simulink model "constraints_comparison_Corsair"  (R2016a)
settings: Solver=ode4  StartTime=0.0  StopTime=30  FixedStep=0.01  RelTol=1e-3
undefined symbols (not defined in the file): acm_aero_model, acm_T_N, breakpoints1, Cm0, Cmde, Cmq, dail, de, dele, drud, Fr_mp_1, Fr_mp_2, Fr_rp_1, Fr_rp_2, ini_acm_de_deg, ini_acm_p_deg_per_s, ini_acm_phi_deg, ini_acm_psi_deg, ini_acm_q_deg_per_s, ini_acm_r_deg_per_s, ini_acm_theta_deg, ini_cmp_de_deg, ini_rig_p_deg_per_s, ini_rig_phi_deg, ini_rig_psi_deg, ini_rig_q_deg_per_s, ini_rig_r_deg_per_s, ini_rig_theta_deg, K1_svo_acm, K1_svo_cmp, K2_svo_acm, K2_svo_cmp, La, Ma, max_defl_sat_acm, max_defl_sat_cmp, max_rate_sat, max_rate_sat_acm, max_rate_sat_cmp, Na, sigbuilder_block, simstop, windspeed, Xa, Ya, Za
libraries: aerolibconvert2 x98, simulink x46, aerolibtransform2 x18
(part 5 of 6)

== matlab function constraints_comparison_Corsair/Equations of motion ==
  data: qa input size=[7,1]; qa_dot_dot output size=[7,1]; qa_dot input size=[7,1]; qa_dot_dot2 input size=[7,1]; theta input; phi input; dail input size=[1,1]; dele input size=[1,1]; drud input size=[1,1]; thrust input; Fa output size=[3,1]; V output; corsair_long output size=[3,1]; corsair_lat output
function [qa_dot_dot, Fa, V, corsair_long,corsair_lat] = fcn(qa, qa_dot, qa_dot_dot2,theta,phi, dail, dele, drud, thrust)

%% Choose constraint type:
% 1 = unconstrained
% 2 = spherical constraint
% 3 = planar constraint

cons = 1;

%% Constants
g = 9.81*0;

% %% Aircraft properties (Hawk)
% 
% m_a = 1.970; % 1.645; % kg
% Ixx_a = 0.008083; % 0.00959; % kg.m^2
% Iyy_a = 0.038; %0.047642; % 0.044; % kg.m^2
% Izz_a = 0.061206; % 0.0507; % kg.m^2
% Ixy_a = 0; % kg.m^2
% Ixz_a = 0; % kg.m^2
% Iyz_a = 0; % kg.m^2
% 
% % Position of body axes origin (c.g. position) relative to inertial axes origin in body frame of reference
% ua0 = [ 0.8*0
%         0.0
%         0.0  ];

%% Aircraft properties (Corsair, taken from Aircraft Stability and Control Data, Gary L. Teper, 1969)

% m_a = 9928.6834; % kg
% Ixx_a = 18486.5777; % kg.m^2
% Iyy_a = 79947.1611; % kg.m^2
% Izz_a = 91599.0606; % kg.m^2
% Ixy_a = 0; % kg.m^2
% Ixz_a = 0; % kg.m^2
% Iyz_a = 0; % kg.m^2

% DC-8
m_a = 86104.03; % kg
Ixx_a = 4216593.82; % kg.m^2
Iyy_a = 3986104.77; % kg.m^2
Izz_a = 7972209.54; % kg.m^2
Ixy_a = -87450.2577; % kg.m^2
Ixz_a = 0; % kg.m^2
Iyz_a = 0; % kg.m^2

% Position of body axes origin (c.g. position) relative to inertial axes origin in body frame of reference
ua0 = [ 0.8*0
        0.0
        0.0  ];
    
%% Input position and attitude vectors

Ra1 = qa(1);
Ra2 = qa(2);
Ra3 = qa(3);
qa0 = qa(4);
qa1 = qa(5);
qa2 = qa(6);
qa3 = qa(7);

%% Input linear and angular velocity vectors

Ra1_dot = qa_dot(1);
Ra2_dot = qa_dot(2);
Ra3_dot = qa_dot(3);
qa0_dot = qa_dot(4);
qa1_dot = qa_dot(5);
qa2_dot = qa_dot(6);
qa3_dot = qa_dot(7);

%% Transformation matrices
            
Ea = [  -qa1     qa0      -qa3     qa2
        -qa2     qa3      qa0      -qa1
        -qa3     -qa2     qa1      qa0  ];
    
E_dasha = [     -qa1     qa0      qa3      -qa2
                -qa2     -qa3     qa0      qa1
                -qa3     qa2      -qa1     qa0  ];
            
Aa = Ea*transpose(E_dasha);

%% Mass and inertial matrix (M) of system
        
% Mass matrix of aircraft model
Ma_RR = [   m_a	0   0
            0   m_a	0
            0   0   m_a	];
        
% Inertial tensor of aircraft model in body frame of reference about c.g./body axes
Ia = [   Ixx_a	-Ixy_a	-Ixz_a
        -Ixy_a	 Iyy_a	-Iyz_a
        -Ixz_a	-Iyz_a	 Izz_a	];
    
MMa = [  Ma_RR    	zeros(3,4)
        zeros(4,3)	transpose(2*E_dasha)*Ia*2*E_dasha	];
    
M = [   MMa  	];

%% Aerodynamics model

rho = 1.225;%1.218; % Density (kg/m^3)
% rho = 1.218; % Density (kg/m^3) Bristol

V_t = 96.6216; %30; % Tunnel windspeed (m/s)

% Calculating angle of attack (alpha), sideslip (sideslip) and local angular velocities (p, q, r)

% Velocity of aircraft in inertial axes
V_a_dot_inertial = [    qa_dot(1)+V_t
                        qa_dot(2)
                        qa_dot(3)      ];
                    
V_a_dot_inertial_pert = [  	qa_dot(1)
                            qa_dot(2)
                            qa_dot(3)      ];
                    
% Acceleration of aircraft in inertial axes (total accelerations is the same are perturbation accelerations)
V_a_dot_dot_inertial_pert = [ 	qa_dot_dot2(1)
                                qa_dot_dot2(2)
                                qa_dot_dot2(3)   ];

% Velocity of aircraft in body axes (vector_inertial = A * vector_body, where A is the transformation matrix)
V_a_dot_body = transpose(Aa)*V_a_dot_inertial;
V_a_dot_body_pert = transpose(Aa)*V_a_dot_inertial_pert;

% Acceleration of aircraft in body axes (vector_inertial = A * vector_body, where A is the transformation matrix)
V_a_dot_dot_body_pert = transpose(Aa)*V_a_dot_dot_inertial_pert;

% Magnitude of total local velocity vector
V = sqrt((V_a_dot_inertial(1))^2+(V_a_dot_inertial(2))^2+(V_a_dot_inertial(3))^2);

% Angle of attack (alpha)
alpha = atan2(V_a_dot_body(3),V_a_dot_body(1));

% Sideslip angle (beta)
beta = asin(V_a_dot_body(2)/V);

% Local angular velocities (p, q, r in body axes)
omega_dasha = 2*E_dasha*[	qa0_dot
                            qa1_dot
                            qa2_dot
                            qa3_dot     ];

p = omega_dasha(1);
q = omega_dasha(2);
r = omega_dasha(3);

% % Reference dimensions (Hawk)
% c = 0.143;        % m
% S = 0.084942;     % m^2
% b = 0.594;        % m
% Reference dimensions (Corsair, taken from Aircraft Stability and Control Data, Gary L. Teper, 1969)
c = 3.29184;      	% m
S = 33.1664;     	% m^2
b = 11.79576;     	% m

% Reference dimensions (Corsair, taken from Aircraft Stability and Control Data, Gary L. Teper, 1969)
c2 = 3.29184;      	% m
S2 = 33.1664;     	% m^2
b2 = 11.79576;     	% m

% A-7A Corsair II (taken from Aircraft Stability and Control Data, Gary L. Teper, 1969)
% Flight conditions: 15,000 ft at Mach 0.3 (no. 4 in reference)
% Initial angle of attack = 13.3 deg
% Initial elevator deflection = -8.8 deg

rho2 = 0.77100671563;	% kg/m^3 (0.001496 slugs/ft^3)
qbar = 367.6468;        % kg/m^2 (75.3 lb/ft^2)
VT0 = 96.6216;          % m/s (317 ft/sec)
U0 = 94.1832;           % m/s (309 ft/sec)

m_a2 = 9928.6834;       % kg
Ixx_a2 = 18486.5777;    % kg.m^2
Iyy_a2 = 79947.1611; 	% kg.m^2
Izz_a2 = 91599.0606; 	% kg.m^2

% Longitudinal dimensional derivatives (body axes, taken from Aircraft Stability and Control Data, Gary L. Teper, 1969)
% X_w     =   0.00464;    % 1/s
% X_u     =   0.00501;    % 1/s
% X_dele  =   5.63;       % ft/(s^2 rad)
% Z_w     =   -0.545;     % 1/s
% Z_u     =   -0.0857;    % 1/s
% Z_dele  =   -23.8;      % ft/(s^2 rad)
% M_w     =   -0.00777;   % 1/(s ft)
% M_w_dot =   -0.000178;  % 1/(s ft)
% M_q     =   -0.340;     % 1/s
% M_u     =   0.00183;    % 1/(s ft)
% M_dele  =   -4.52;      % 1/s^2
% Longitudinal dimensional derivatives (body axes, taken from Cook page 148)
% X_q     =   -72.9;      % ft/s
% X_theta =   -31.34;     % ft/(s^2 rad)
% Z_q     =   309.0;      % ft/s
% Z_theta =   -7.4;       % ft/(s^2 rad)
% M_q see above
% M_theta =   0.00132;    % 1/s^2

% Units conversion
X_u     =   0.00501;                    % 1/s
X_w     =   0.00464;                    % 1/s
X_q     =   -72.9*0.3048;               % m/s
X_theta =   -31.34*0.3048;              % m/(s^2 rad)
X_dele  =   5.63*0.3048;                % m/(s^2 rad)
Z_u     =   -0.0857;                    % 1/s
Z_w     =   -0.545;                     % 1/s
Z_q     =   309.0*0.3048;               % m/s
Z_theta =   -7.4*0.3048;                % m/(s^2 rad)
Z_dele  =   -23.8*0.3048;               % m/(s^2 rad)
M_u     =   0.00183*(1/0.3048);         % 1/(s m)
M_w     =   -0.00777*(1/0.3048);        % 1/(s m)
% M_w_dot =   -0.000178*(1/0.3048);       % 1/(s m)
M_q     =   -0.340*0-0.395;            	% 1/s
M_theta =   0.00132;                    % 1/s^2
M_dele  =   -4.52;                      % 1/s^2

% % % % Longitudinal dimensional derivatives (body axes, taken from Aircraft Stability and Control Data, Gary L. Teper, 1969)
% % % % Y_v     =   -0.122;       % 1/s
% % % % Y_dail  =   -0.00150;     % ft/(s^2)
% % % % Y_drud  =   0.0307;       % ft/(s^2)
% % % % L_beta  =   -8.79;        % 1/s^2
% % % % L_p     =   -1.38;        % 1/s
% % % % L_r     =   0.857;        % 1/s
% % % % L_dail  =   3.75;         % 1/s^2
% % % % L_drud  =   1.82;         % 1/s^2
% % % % N_beta  =   0.948;        % 1/s^2 
% % % % N_p     =   -0.0310;      % 1/s
% % % % N_r     =   -0.271;       % 1/s     
% % % % N_dail  =   0.280;        % 1/s^2
% % % % N_rud   =   -1.56;        % 1/s^2
% % % 
% % % % Units conversion
% % % Y_v     =   -0.122;             % 1/s
% % % Y_dail  =   -0.00150*0.3048;   	% m/(s^2)
% % % Y_drud  =   0.0307*0.3048;     	% m/(s^2)
% % % L_beta  =   -8.79;              % 1/s^2
% % % L_p     =   -1.38;              % 1/s
% % % L_r     =   0.857;              % 1/s
% % % L_dail  =   3.75;               % 1/s^2
% % % L_drud  =   1.82;               % 1/s^2
% % % N_beta  =   0.948;              % 1/s^2
% % % N_p     =   -0.0310;            % 1/s
% % % N_r     =   -0.271;             % 1/s
% % % N_dail  =   0.280;              % 1/s^2
% % % N_drud   =   -1.56;              % 1/s^2

% Longitudinal dimensional derivatives (body axes, taken from Aircraft Stability and Control Data, Gary L. Teper, 1969)
% Y_v     =   -0.122;       % 1/s
% Y_dail  =   -0.00150;     % ft/(s^2)
% Y_drud  =   0.0307;       % ft/(s^2)
% L_beta  =   -8.79;        % 1/s^2
% L_p     =   -1.38;        % 1/s
% L_r     =   0.857;        % 1/s
% L_dail  =   3.75;         % 1/s^2
% L_drud  =   1.82;         % 1/s^2
% N_beta  =   0.948;        % 1/s^2 
% N_p     =   -0.0310;      % 1/s
% N_r     =   -0.271;       % 1/s     
% N_dail  =   0.280;        % 1/s^2
% N_rud   =   -1.56;        % 1/s^2
% Lateral dimensional derivatives (body axes, taken from Cook page 185)
% Y_phi   =   32.2;         % ft/(s^2 rad)
% Y_r     =   -468.2;       % ft/s

% Units conversion
Y_v     =   -0.1008;                                % 1/s
Y_phi   =   32.2*0.3048;                            % m/(s^2 rad)
Y_r     =   -468.2*0.3048;                          % m/s
Y_dail  =   0*0.3048;                               % m/(s^2)
Y_drud  =   13.48416*0.3048;                        % m/(s^2)
L_v     =   -2.6826/(468.2*0.3048); %-2.71/468.2;  	% 1/s^2
L_p     =   -1.2332; %-1.232;                       % 1/s
L_r     =   0.3913; %0.397;                         % 1/s
L_dail  =   -1.62;                                  % 1/s^2
L_drud  =   0.392;                                  % 1/s^2
N_v     =   1.2710/(468.2*0.3048); %1.301/468.2; 	% 1/s^2
N_p     =   -0.0481; %-0.0346;                    	% 1/s
N_r     =   -0.2524; %-0.257;                       % 1/s
N_dail  =   -0.0365; %-0.01875;                     % 1/s^2
N_drud  =   -0.8602; %-0.864;                       % 1/s^2

% Body axis velocities (p, q, r are already defined above)
u = V_a_dot_body_pert(1);
v = V_a_dot_body_pert(2);
w = V_a_dot_body_pert(3);
% w_dot = V_a_dot_dot_body_pert(3);

% % % % Converting to nondimensional derivatives (see Aircraft Stability and Control Data, Gary L. Teper, 1969)
% % % CX_w     =   X_w*(2*m_a2)/(rho2*S2*U0);
% % % CX_u     =   X_u*(m_a2)/(rho2*S2*U0);
% % % CX_dele  =   -X_dele*(2*m_a2)/(rho2*S2*VT0^2);
% % % CZ_w     =   Z_w*(2*m_a2)/(rho2*S2*U0);
% % % CZ_u     =   Z_u*(m_a2)/(rho2*S2*U0);
% % % CZ_dele  =   -Z_dele*(2*m_a2)/(rho2*S2*VT0^2);
% % % CM_w     =   M_w*(2*Iyy_a2)/(rho2*S2*c2*U0);
% % % CM_w_dot =   M_w_dot*(4*Iyy_a2*VT0)/(rho2*S2*c2^2*U0);
% % % CM_q     =   M_q*(4*Iyy_a2)/(rho2*S2*c2^2*VT0);
% % % CM_u     =   M_u*(2*Iyy_a2)/(rho2*S2*c2*U0);
% % % CM_dele  =   M_dele*(2*Iyy_a2)/(rho2*S2*c2*VT0);
% % % 
% % % CX = -(CX_w*w + CX_u*u + CX_dele*dele); % Negative because Teper sign convention is positive aft
% % % CZ = CZ_w*w + CZ_u*u + CZ_dele*dele;
% % % % CM = CM_w*w + CM_w_dot*w_dot + CM_q*q + CM_u*u + CM_dele*dele;
% % % CM = CM_w*w + CM_q*q + CM_u*u + CM_dele*dele;
% % % 
% % % CY = 0;
% % % CL = 0;
% % % CN = 0;

X_body = m_a*X_w*w + m_a*X_u*u + m_a*X_dele*dele + m_a*X_q*q + m_a*X_theta*theta;
Y_body = m_a*Y_v*v + m_a*Y_dail*dail + m_a*Y_drud*drud + m_a*Y_phi*phi + m_a*Y_r*r;
Z_body = m_a*Z_w*w + m_a*Z_u*u + m_a*Z_dele*dele + m_a*Z_q*q + m_a*Z_theta*theta;

L_body = Ixx_a*L_v*v + Ixx_a*L_p*p + Ixx_a*L_r*r + Ixx_a*L_dail*dail + Ixx_a*L_drud*drud;
M_body = Iyy_a*M_w*w + Iyy_a*M_u*u + Iyy_a*M_dele*dele + Iyy_a*M_q*q + Iyy_a*M_theta*theta;
N_body = Izz_a*N_v*v + Izz_a*N_p*p + Izz_a*N_r*r + Izz_a*N_dail*dail + Izz_a*N_drud*drud;
    
% Wind axes forces and moments
% % % X_wind=0.5*rho*V^2*S*CX;
% % % Y_wind=0.5*rho*V^2*S*CY;
% % % Z_wind=0.5*rho*V^2*S*CZ;
% % % 
% % % L_wind=0.5*rho*V^2*S*b*CL;
% % % M_wind=0.5*rho*V^2*S*c*CM;
% % % N_wind=0.5*rho*V^2*S*b*CN;

% X_wind=0.5*rho2*V^2*S*CX;
% Y_wind=0.5*rho2*V^2*S*CY;
% Z_wind=0.5*rho2*V^2*S*CZ;
% 
% L_wind=0.5*rho2*V^2*S*b*CL;
% M_wind=0.5*rho2*V^2*S*c*CM;
% N_wind=0.5*rho2*V^2*S*b*CN;

% F_wind = [  X_wind
%             Y_wind
%             Z_wind   ];
%         
% M_wind = [  L_wind
%             M_wind
%             N_wind   ];
        
% Body to wind axes transformation
% According to Cook (page 21): (phi,theta,psi) = (0,alpha,-beta)
phi_w = 0;
theta_w = alpha;
psi_w = -beta;

% From NASA transformation equations:
theta1 = psi_w;
theta2 = theta_w;
theta3 = phi_w;

q0 = +sin(theta1/2)*sin(theta2/2)*sin(theta3/2)+cos(theta1/2)*cos(theta2/2)*cos(theta3/2);
q1 = -sin(theta1/2)*sin(theta2/2)*cos(theta3/2)+sin(theta3/2)*cos(theta1/2)*cos(theta2/2);
q2 = +sin(theta1/2)*sin(theta3/2)*cos(theta2/2)+sin(theta2/2)*cos(theta1/2)*cos(theta3/2);
q3 = +sin(theta1/2)*cos(theta2/2)*cos(theta3/2)-sin(theta2/2)*sin(theta3/2)*cos(theta1/2);

E = [  -q1     q0      -q3     q2
        -q2     q3      q0      -q1
        -q3     -q2     q1      q0  ];
    
E_dash = [     -q1     q0      q3      -q2
                -q2     -q3     q0      q1
                -q3     q2      -q1     q0  ];
            
A_b2w = E*transpose(E_dash); % Note: this matrx transforms from body to wind axes!

% Body axes forces and moments
% F_dash_a = transpose(A_b2w)*F_wind + [thrust;0;0];
% M_dash_a = transpose(A_b2w)*M_wind;
F_dash_a = [X_body*0;Y_body;Z_body*0] + [thrust;0;0];
M_dash_a = [L_body;M_body*0;N_body];

% Inertial axes moments
F_a = Aa*F_dash_a;

%% Computing external forces matrix QE
                
% Angular velocity of aircraft model in body frame of reference
omega_dasha = 2*E_dasha*[	qa0_dot
                            qa1_dot
                            qa2_dot
                            qa3_dot     ];
                        
% External translational/linear forces on aircraft model in inertial frame of reference
% Fa1 = 0;
% Fa2 = 0;
% Fa3 = m_a*9.81;
Fa1 = F_a(1);
Fa2 = F_a(2);
Fa3 = F_a(3)+m_a*g;
Fa = [  Fa1
        Fa2
        Fa3    ];
% External moments on aircraft model in body frame of reference
% Ma1 = 0;
% Ma2 = 0;
% Ma3 = 0;
Ma1 = M_dash_a(1);
Ma2 = M_dash_a(2);
Ma3 = M_dash_a(3);
Ma = [  Ma1
        Ma2
        Ma3     ];

QE_a = [    Fa
            transpose(2*E_dasha)*(Ma-cross(omega_dasha,Ia*omega_dasha))	];
        
QE = [  QE_a    ];

%% Solving equations of motion

switch cons
    case 1 % Unconstrained
        
        % Quaternion constriant
        Cq_1 = [	zeros(1,3)	qa0   qa1   qa2   qa3  ];
        QC_1 = -((qa0_dot)^2+(qa1_dot)^2+(qa2_dot)^2+(qa3_dot)^2);
        
        Cq = Cq_1;
        QC = QC_1;
        
    case 2 % Spherical constraint
        
        % Quaternion constriant
        Cq_1 = [	zeros(1,3)	qa0   qa1   qa2   qa3  ];
        QC_1 = -((qa0_dot)^2+(qa1_dot)^2+(qa2_dot)^2+(qa3_dot)^2);
        
        % Spherical constraint
        r = 0.8; % Sphere radius (m)
        Cq_2 = [    (Ra1-r)   Ra2     Ra3     0   0   0   0];
        QC_2 = -Ra1_dot^2 - Ra2_dot^2 - Ra3_dot^2;
        
        Cq = [  Cq_1
                Cq_2  ];
        QC = [  QC_1
                QC_2  ];
        
    case 3 % Planar constraint
        
        % Quaternion constriant
        Cq_1 = [	zeros(1,3)	qa0   qa1   qa2   qa3  ];
        QC_1 = -((qa0_dot)^2+(qa1_dot)^2+(qa2_dot)^2+(qa3_dot)^2);
        
        % Planar constraint
        Cq_2 = [    1   0   0   0   0   0   0   ];
        QC_2 = 0;
        
        Cq = [  Cq_1
                Cq_2  ];
        QC = [  QC_1
                QC_2  ];
            
    case 4 % x and z constriant for validating lateral aerodynamics model
        
        % Quaternion constriant
        Cq_1 = [	zeros(1,3)	qa0   qa1   qa2   qa3  ];
        QC_1 = -((qa0_dot)^2+(qa1_dot)^2+(qa2_dot)^2+(qa3_dot)^2);
        
        % x constraint
        Cq_2 = [    1   0   0   0   0   0   0   ];
        QC_2 = 0;
        
     	% x constraint
        Cq_3 = [    0   0   1   0   0   0   0   ];
        QC_3 = 0;
        
        Cq = [  Cq_1
                Cq_2
                Cq_3  ];
        QC = [  QC_1
                QC_2
                QC_3  ];
        
end

        
MM = [  M   transpose(Cq)
        Cq  zeros(size(QC,1))        ];
QQ = [  QE
        QC  ];

qq = MM\QQ;

%% Output acceleration vectors

qa_dot_dot = qq(1:7);

%% Output for comparing with Cook Corsair model (For theta_a, see output from quaternion converison block)
uu_a        = qa_dot(1)*3.28084; % ft/sec
vv_a        = qa_dot(2)*3.28084; % ft/sec
ww_a        = qa_dot(3)*3.28084; % ft/sec
pp_a        = p;                 % rad/s
qq_a        = q;                 % rad/s
rr_a        = r;                 % rad/s

corsair_long = [ uu_a
                 ww_a
                 qq_a ];
             
corsair_lat  = [ vv_a
                 pp_a
                 rr_a ];

== matlab function constraints_comparison_Corsair/Subsystem14/Subsystem13/MATLAB Function ==
  data: q input; x_ini output; y_ini output; z_ini output
function [x_ini,y_ini,z_ini]= fcn(q)

% Initial position

x = 0.8;
z = 0.1433;%0.03975;

p = [   x
        0
        z   ];

q0 = q(1);
q1 = q(2);
q2 = q(3);
q3 = q(4);

E = [  -q1     q0      -q3     q2
       -q2     q3      q0      -q1
       -q3     -q2     q1      q0  ];
    
E_dash = [     -q1     q0      q3      -q2
               -q2     -q3     q0      q1
               -q3     q2      -q1     q0  ];
           
A = E*transpose(E_dash);

p_in = A*p;

x_ini = p_in(1);
y_ini = p_in(2);
z_ini = p_in(3);

== matlab function constraints_comparison_Corsair/Subsystem14/Aircraft acceleration body axis ==
  data: Aa input; qa_dot_dot3 output; qa_dot_dot2 input; nz output
function [qa_dot_dot3,nz]= fcn(Aa, qa_dot_dot2)

% qa_dot_dot2 = linear accelerations in inertial frame
% qa_dot_dot3 = linear accelerations in body axis

qa_dot_dot3 = Aa\qa_dot_dot2;
% qa_dot_dot3 = qa_dot_dot2;

theta_acm = atan(-Aa(3,1)/sqrt(1-(Aa(3,1))^2));
nz = qa_dot_dot2(3)*cos(theta_acm)-qa_dot_dot2(1)*sin(theta_acm);

== matlab function constraints_comparison_Corsair/Subsystem14/Aerodynamics model: compensator ==
  data: qc input; V_t input; alpha input; beta input; q input; eta input; F_c output; M_dash_c output; r input; rudd input; extra output
function [F_c,M_dash_c,extra] = fcn(qc,V_t,alpha,beta,q,eta,r,rudd)

% beta = 0;

Rc1 = qc(1);
Rc2 = qc(2);
Rc3 = qc(3);
qc0 = qc(4);
qc1 = qc(5);
qc2 = qc(6);
qc3 = qc(7);

% Transformation matrices
Ec = [  -qc1     qc0      -qc3     qc2
        -qc2     qc3      qc0      -qc1
        -qc3     -qc2     qc1      qc0  ];
    
E_dashc = [     -qc1     qc0      qc3      -qc2
                -qc2     -qc3     qc0      qc1
                -qc3     qc2      -qc1     qc0  ];

Ac = Ec*transpose(E_dashc);

% Reference dimensions
c = 0.181;      % m
S = 0.1254;     % m^2
b = 0.7;        % m

% % Control surface deflection
% eta = dcs(1); % Virtual ailerons
% eta = dcs(2); % Virtual elevator
% eta = dcs(3); % Virtual rudder

% Aerodynamic coefficients (alpha = theta_rig)
% CL=3.647*alpha+1.306*eta+(2.302*0.181/V_t)*q; % Pattinson
% CL=2.18*alpha+0.5*eta+(b*15/(2*V_t))*q; % Matthew (old)
CL=1.73*alpha+1.42*eta+(b*4.69/(2*V_t))*q; % Matthew (13th Oct 2015)
% CD=CL^2/(3.907*pi); % Pattinson
CD=0; % Matthew
CM=0; % Pattinson/Matthew

% Side force
CY = 1.73*-beta+1.42*rudd+(b*4.69/(2*V_t))*r;

% Dynamic pressure
rho = 1.225;% 1.218; % Density (kg/m^3)
Dyn_p = 0.5*rho*V_t^2;

% Loads in wind axes (relative to total local velocity vector)
L = Dyn_p*S*CL;
D = Dyn_p*S*CD;
M = Dyn_p*S*c*CM;

Y = Dyn_p*S*CY;

% Transforming loads to body frame of reference from wind axes (See Cook p.21)
phi = 0;
theta = alpha;
psi = -beta;

% q0 = cos(phi/2)*cos(theta/2)*cos(psi/2)+sin(phi/2)*sin(theta/2)*sin(psi/2);
% q1 = cos(phi/2)*cos(theta/2)*sin(psi/2)-sin(phi/2)*sin(theta/2)*cos(psi/2);
% q2 = cos(phi/2)*sin(theta/2)*cos(psi/2)+sin(phi/2)*cos(theta/2)*sin(psi/2);
% q3 = sin(phi/2)*cos(theta/2)*cos(psi/2)-cos(phi/2)*sin(theta/2)*sin(psi/2);
% 
% E = [  -q1     q0      -q3     q2
%         -q2     q3      q0      -q1
%         -q3     -q2     q1      q0  ];
%     
% E_dash = [     -q1     q0      q3      -q2
%                 -q2     -q3     q0      q1
%                 -q3     q2      -q1     q0  ];
%             
% A = E*transpose(E_dash);

theta1 = psi;
theta2 = theta;
theta3 = phi;

q0 = +sin(theta1/2)*sin(theta2/2)*sin(theta3/2)+cos(theta1/2)*cos(theta2/2)*cos(theta3/2);
q1 = -sin(theta1/2)*sin(theta2/2)*cos(theta3/2)+sin(theta3/2)*cos(theta1/2)*cos(theta2/2);
q2 = +sin(theta1/2)*sin(theta3/2)*cos(theta2/2)+sin(theta2/2)*cos(theta1/2)*cos(theta3/2);
q3 = +sin(theta1/2)*cos(theta2/2)*cos(theta3/2)-sin(theta2/2)*sin(theta3/2)*cos(theta1/2);

E = [	-q1     q0      -q3     q2
        -q2     q3      q0      -q1
        -q3     -q2     q1      q0  ];
    
E_dash = [	-q1     q0      q3      -q2
           	-q2     -q3     q0      q1
           	-q3     q2      -q1     q0  ];
            
A10 = E*transpose(E_dash);
A10_transpose_inertial_to_body = A10';

F_dash_c = A10_transpose_inertial_to_body*[ -D
                                            Y
                                            -L  ];
                      
% M_dash_c = transpose(A)*[ 0
%                           M
%                           0   ];
M_dash_c = A10_transpose_inertial_to_body*[  0
                                             M
                                             0   ];
                    
% Transforming forces onto inertial frame
F_c = Ac*F_dash_c;

% F_c = [     -D*0
%             0
%             -L  ]; %/cos(alpha)

% F_c = zeros(3,1);
% M_dash_c = zeros(3,1);

%% Extra
extra = [   alpha*180/pi
            beta*180/pi
            -D
            Y
            -L
            F_dash_c
            F_c];

== matlab function constraints_comparison_Corsair/Subsystem14/MATLAB Function7 ==
  data: V_t output size=[1]; qc input size=[7,1]; theta_rig output size=[1]; p output; qc_dot input size=[7,1]; q output size=[1]; r output; qc_dot_dot input; Vt input; Vc output; omega_dashc_dot output
function [V_t,theta_rig,p,q,r,Vc,omega_dashc_dot] = fcn(qc,qc_dot,qc_dot_dot,Vt)
  
Rc1 = qc(1);
Rc2 = qc(2);
Rc3 = qc(3);
qc0 = qc(4);
qc1 = qc(5);
qc2 = qc(6);
qc3 = qc(7);

Rc1_dot = qc_dot(1);
Rc2_dot = qc_dot(2);
Rc3_dot = qc_dot(3);
qc0_dot = qc_dot(4);
qc1_dot = qc_dot(5);
qc2_dot = qc_dot(6);
qc3_dot = qc_dot(7);

Rc1_dot_dot = qc_dot_dot(1);
Rc2_dot_dot = qc_dot_dot(2);
Rc3_dot_dot = qc_dot_dot(3);
qc0_dot_dot = qc_dot_dot(4);
qc1_dot_dot = qc_dot_dot(5);
qc2_dot_dot = qc_dot_dot(6);
qc3_dot_dot = qc_dot_dot(7);

% Transformation matrices
Ec = [  -qc1     qc0      -qc3     qc2
        -qc2     qc3      qc0      -qc1
        -qc3     -qc2     qc1      qc0  ];
    
E_dashc = [     -qc1     qc0      qc3      -qc2
                -qc2     -qc3     qc0      qc1
                -qc3     qc2      -qc1     qc0  ];

Ac = Ec*transpose(E_dashc);

% Wind tunnel velocity vector
Vtt = [  Vt
         0   
         0   ];

% Velocity vector of aircraft model in inertial frame of reference
Vc = [  Rc1_dot
        Rc2_dot
        Rc3_dot	];

% Total velocity vector of aircraft model in body frame of reference
Vc_dash = transpose(Ac)*(Vc + Vtt);

% Magnitude of total local velocity vector
V0 = sqrt((Vc_dash(1))^2+(Vc_dash(2))^2+(Vc_dash(3))^2);

% Angle of attack
alpha = atan2(Vc_dash(3),Vc_dash(1));

% Acceleration in body frame
c_dash = transpose(Ac)*[    Rc1_dot_dot
                            Rc2_dot_dot
                            Rc3_dot_dot     ];

% Acceleration in z-direction body frame
w_dot = c_dash(3);

% Sideslip angle [CHECK SIGN]
beta = asin(Vc_dash(2)/V0);

% Local angular velocities
omega_dashc = 2*E_dashc*[	qc0_dot
                            qc1_dot
                            qc2_dot
                            qc3_dot     ];
                        
% Angular rate
p = omega_dashc(1); % rad/s
q = omega_dashc(2); % rad/s
r = omega_dashc(3); % rad/s

V_t = Vtt(1);

% Rig pitch angle
% theta_rig = atan2(-Ac(3,1),sqrt(1-(Ac(3,1))^2));
theta_rig = 0;

%% Local angular acceleration
omega_dashc_dot = 2*E_dashc*[	qc0_dot_dot
                            qc1_dot_dot
                            qc2_dot_dot
                            qc3_dot_dot     ];

== matlab function constraints_comparison_Corsair/Subsystem14/Aerodynamics model: Hawk ==
  data: Cm0 input; Cmde input; de input; Cmq input; T input; acm_aero_model input; qa input; V0 input; alpha input; w_dot input; q input; eta input; F_a output; M_dash_a output; q_rig input; Aa output
function [F_a,M_dash_a,Aa] = fcn(Cm0,Cmde,de,Cmq,T,acm_aero_model,qa,V0,alpha,w_dot,q,eta,q_rig)

beta = 0;

Ra1 = qa(1);
Ra2 = qa(2);
Ra3 = qa(3);
qa0 = qa(4);
qa1 = qa(5);
qa2 = qa(6);
qa3 = qa(7);

% Transformation matrices
Ea = [  -qa1     qa0      -qa3     qa2
        -qa2     qa3      qa0      -qa1
        -qa3     -qa2     qa1      qa0  ];
    
E_dasha = [     -qa1     qa0      qa3      -qa2
                -qa2     -qa3     qa0      qa1
                -qa3     qa2      -qa1     qa0  ];

Aa = Ea*transpose(E_dasha);

% Reference dimensions (Hawk)
c = 0.143;       % m
S = 0.084942;    % m^2

% theta_acm = atan(-Aa(3,1)/sqrt(1-(Aa(3,1))^2));
% aplha_approx = theta_acm -0.8*q_rig/30;

% Aerodynamic coefficients
% (Note: CL0=0.1155 is multiplied by a factor of 1.80 to match experimental
%  data)
% CL=0.1155*1.80/1.80+3.8004*alpha+0.4429*eta-0.4456*alpha*eta-4.447*alpha^2-0.04322*eta^2-7.314*alpha*eta^2-4.636*alpha^2*eta+0.0008039*alpha^3+0.001499*eta^3+1.828*q*c/V0*0+33*(c/(2*V0))*q+1.342*c/(V0^2)*w_dot*0;
% CD=0.04953+0.04801*alpha-0.008018*eta+0.4703*alpha*eta+1.669*alpha^2+0.3445*eta^2+0.2102*alpha*eta^2-0.9875*alpha^2*eta+0.00001016*alpha^3-0.00002714*eta^3;
% CM=0.04463-0.5919*alpha-0.7774*eta+0.4383*alpha*eta-0.1227*alpha^2-0.4214*eta^2-2.587*alpha*eta^2+3.292*alpha^2*eta-0.0001252*alpha^3-0.002631*eta^3-3.528*q*c/V0-2.604*c/(V0^2)*w_dot*0;

% CL=0.1155*0.75+3.8004*0.75*alpha+0.4429*0.75*eta-0.4456*alpha*eta-4.447*alpha^2-0.04322*eta^2-7.314*alpha*eta^2-4.636*alpha^2*eta+0.0008039*alpha^3+0.001499*eta^3-1.828*q*c/V0-1.342*c/(V0^2)*w_dot;
% CD=0.04953*0.75+0.04801*0.75*alpha-0.008018*0.75*eta+0.4703*alpha*eta+1.669*alpha^2+0.3445*eta^2+0.2102*alpha*eta^2-0.9875*alpha^2*eta+0.00001016*alpha^3-0.00002714*eta^3;
% CM=0.04463*0.75-0.5919*0.75*alpha-0.7774*0.75*eta+0.4383*alpha*eta-0.1227*alpha^2-0.4214*eta^2-2.587*alpha*eta^2+3.292*alpha^2*eta-0.0001252*alpha^3-0.002631*eta^3-3.528*q*c/V0-2.604*1/(V0^2)*w_dot

% CL = 0.1155*1.80 + 3.8*alpha + 0.4431009*eta + 33*(c/(2*V0))*q; % Linear model (Matthew)
% CD=0.04953+0.04801*alpha-0.008018*eta+0.4703*alpha*eta+1.669*alpha^2+0.3445*eta^2+0.2102*alpha*eta^2-0.9875*alpha^2*eta+0.00001016*alpha^3-0.00002714*eta^3;
% CD=0.04953+0.04801*alpha+1.669*alpha^2; % Simplified
% CM = Cm0 + Cmde*(eta-de) + Cmq*(c/(2*V0))*q; % Matthew's data (13th Oct 2015)

% V0 = 30;%%%%
% alpha2 = (theta_acm - 0.8*q_rig/30);%%%%

switch acm_aero_model
    case 1 % Nanjing
        CL=0.1155+3.8004*alpha+0.4429*eta-0.4456*alpha*eta-4.447*alpha^2-0.04322*eta^2-7.314*alpha*eta^2-4.636*alpha^2*eta+0.0008039*alpha^3+0.001499*eta^3-1.828*q*c/V0-1.342*c/(V0^2)*w_dot;
        CD=0.04953+0.04801*alpha-0.008018*eta+0.4703*alpha*eta+1.669*alpha^2+0.3445*eta^2+0.2102*alpha*eta^2-0.9875*alpha^2*eta+0.00001016*alpha^3-0.00002714*eta^3;
        CM=0.04463-0.5919*alpha-0.7774*eta+0.4383*alpha*eta-0.1227*alpha^2-0.4214*eta^2-2.587*alpha*eta^2+3.292*alpha^2*eta-0.0001252*alpha^3-0.002631*eta^3-3.528*q*c/V0-2.604*1/(V0^2)*w_dot;
    case 2 % Matthew's linear model
        CL = 0.1155*1.80 + 3.8*alpha + 0.4431009*eta + 33*(c/(2*V0))*q;
        CD = 0;
        CM = 0.04463 -0.528*alpha -8.14*(c/(2*V0))*q -0.84*eta;
    case 3 % Matthew's linear model + lookup table for CM
        CL = 0.1155*1.80 + 3.8*alpha + 0.4431009*eta + 33*(c/(2*V0))*q;
        CD = 0;
        CM = Cm0 + Cmde*(eta-de) + Cmq*(c/(2*V0))*q; % Matthew's data (13th Oct 2015)
    otherwise
        CL = 0;
        CD = 0;
        CM = 0;
end

% Dynamic pressure
rho = 1.225;%1.218; % Density (kg/m^3)
Dyn_p = 0.5*rho*V0^2;

% Loads in wind axes (relative to total local velocity vector)
L = Dyn_p*S*CL;
D = Dyn_p*S*CD;
M = Dyn_p*S*c*CM;

% Transforming loads to body frame of reference from wind axes (See Cook p.21, rotation sequence: 0->3 YAW, PITCH, ROLL)
phi = 0;
theta = alpha;
psi = -beta;

% q0 = cos(phi/2)*cos(theta/2)*cos(psi/2)+sin(phi/2)*sin(theta/2)*sin(psi/2);
% q1 = cos(phi/2)*cos(theta/2)*sin(psi/2)-sin(phi/2)*sin(theta/2)*cos(psi/2);
% q2 = cos(phi/2)*sin(theta/2)*cos(psi/2)+sin(phi/2)*cos(theta/2)*sin(psi/2);
% q3 = sin(phi/2)*cos(theta/2)*cos(psi/2)-cos(phi/2)*sin(theta/2)*sin(psi/2);

theta1 = psi;
theta2 = theta;
theta3 = phi;

q0 = +sin(theta1/2)*sin(theta2/2)*sin(theta3/2)+cos(theta1/2)*cos(theta2/2)*cos(theta3/2);
q1 = -sin(theta1/2)*sin(theta2/2)*cos(theta3/2)+sin(theta3/2)*cos(theta1/2)*cos(theta2/2);
q2 = +sin(theta1/2)*sin(theta3/2)*cos(theta2/2)+sin(theta2/2)*cos(theta1/2)*cos(theta3/2);
q3 = +sin(theta1/2)*cos(theta2/2)*cos(theta3/2)-sin(theta2/2)*sin(theta3/2)*cos(theta1/2);

E = [  -q1     q0      -q3     q2
        -q2     q3      q0      -q1
        -q3     -q2     q1      q0  ];
    
E_dash = [     -q1     q0      q3      -q2
                -q2     -q3     q0      q1
                -q3     q2      -q1     q0  ];
            
 A = E*transpose(E_dash); % body axes to inertial/wind axes transformation

% Free-flying model thrust (in body axes)
thrust = T; %3.55; %3.126;

F_dash_a2 = transpose(A)*[ -D
                          0
                          -L  ];
                      
F_dash_a = F_dash_a2 + [    thrust
                            0
                            0       ];
                    
M_dash_a = transpose(A)*[ 0
                          M
                          0   ];
                    
% Transforming forces onto inertial frame
F_a = Aa*F_dash_a;

% F_a = [ -D+thrust
%          0
%         -L  ]; % /cos(theta_acm)

% F_a = zeros(3,1);
% M_dash_a = zeros(3,1);

== matlab function constraints_comparison_Corsair/Subsystem14/MATLAB Function8 ==
  data: A3 input; A33 output
function A33 = fcn(A3)

A33 = [ A3(1,1)
        A3(2,1)
        A3(3,1)
        A3(1,2)
        A3(2,2)
        A3(3,2)
        A3(1,3)
        A3(2,3)
        A3(3,3) ];

== matlab function constraints_comparison_Corsair/Subsystem14/Aircraft_model_friction ==
  data: theta_dot_rp input; theta_dot_mp input; Fr_mp output; theta_dot_relative output
function [Fr_mp,theta_dot_relative] = fcn(theta_dot_rp,theta_dot_mp)

theta_dot_relative = theta_dot_mp-theta_dot_rp;

%% John Pattinson's friction model
% Fs_mp = 2.74E-4;
% Fc_mp = 1.68E-3;
% omega2_mp = 3.94E-4;
% 
% Fr_mp = [   0
%             -((sign(theta_dot)*(Fs_mp+Fc_mp)/2 + omega2_mp.*theta_dot))
%             0                                                                   ];
%         
% if abs(theta_dot) < 1E-3
%     Fr_mp = [   0
%             	0
%                 0	];
% end

%% Sergio's friction model (parameter estimation) 09-11-2015
% Model gimbal
k1m = 35.97e-3;
k2m = 0.239e-3;
k3m = 112e3;

Fr_mp = [   0
            -(k1m*theta_dot_relative + k2m*tanh(k3m*theta_dot_relative))
            0                                                                   ];

% if abs(theta_dot) < 1E-3
%     Fr_mp = [   0
%             	0
%                 0	];
% end

== matlab function constraints_comparison_Corsair/Subsystem14/Compensator friction ==
  data: theta_dot_rp input; Fr_rp output
function Fr_rp  = fcn(theta_dot_rp)

%% John Pattinson's friction model
% Fs_rp = 2.79E-2;
% Fc_rp = 3.39E-2;
% omega2_rp = 4.10E-3;
% 
% Fr_rp = [   0
%             -((sign(theta_dot_rp)*(Fs_rp+Fc_rp)/2 + omega2_rp.*theta_dot_rp))
%             0                                                                       ];

%% Sergio's friction model (parameter estimation) 09-11-2015
% Rig gimbal
k1r = 6.324e-3;
k2r = 24.42e-3;
k3r = 25;

Fr_rp = [   0
            -(k1r*theta_dot_rp + k2r*tanh(k3r*theta_dot_rp))
            0                                                                   ];

== matlab function constraints_comparison_Corsair/Subsystem14/Virtual compensator deflections to physical deflections ==
  data: da_cmp input; servo1 output; de_cmp input; dr_cmp input; servo2 output; servo3 output; servo4 output; s2 output; da_cmp2 output; de_cmp2 output; dr_cmp2 output
function [servo1,servo2,servo3,servo4,s2,da_cmp2,de_cmp2,dr_cmp2] = fcn(da_cmp, de_cmp, dr_cmp)

d = [   da_cmp
        de_cmp
        dr_cmp  ];
    
A = [   1    1  -1
        1   -1  -1
        1   -1   1
        1    1   1  ];
    
s = A*d;

servo1 = s(1);
servo2 = s(2);
servo3 = s(3);
servo4 = s(4);

% Limiting servo deflection
if servo1 > 40*pi/180
    servo1 = 40*pi/180;
end
if servo2 > 40*pi/180
    servo2 = 40*pi/180;
end
if servo3 > 40*pi/180
    servo3 = 40*pi/180;
end
if servo4 > 40*pi/180
    servo4 = 40*pi/180;
end

if servo1 < -40*pi/180
    servo1 = -40*pi/180;
end
if servo2 < -40*pi/180
    servo2 = -40*pi/180;
end
if servo3 < -40*pi/180
    servo3 = -40*pi/180;
end
if servo4 < -40*pi/180
    servo4 = -40*pi/180;
end

s2 = [ 	servo1
        servo2
        servo3
        servo4  ];
    
A = [   1    1  -1   1
        1   -1  -1  -1
        1   -1   1  +1
        1    1   1  -1  ];
    
% NOTE: last column on matrix A is redundant to make a square matrix for
% inversion
    
d = A\s2;

da_cmp2 = d(1); % Virtual ailerons not used because direct control surface defections are fed to roll model
de_cmp2 = d(2);
dr_cmp2 = d(3);

== matlab function constraints_comparison_Corsair/Subsystem14/Aircraft attitude relative to arm2 ==
  data: phi_acm output; theta_acm output; psi_acm output; phi_arm output; theta_arm output; psi_arm output; Ar input; Aa input; phi_relative output; qr input; qa input; theta_relative output; psi_relative output
function [phi_acm,theta_acm,psi_acm,phi_arm,theta_arm,psi_arm,phi_relative,theta_relative,psi_relative]= fcn(Ar, Aa, qr, qa)

% qa is the state vector of the aircraft model in the inertial frame
% So, qa in the aircraft model's body frame is:

% qa_b = Aa\qa(4:7,1);

% A = Aa/Ar; % [CORRECT]

% A = Ar/Aa; [WRONG]
A = transpose(Ar)*Aa; % [CORRECT]

% A = Ar*inv(Aa);


% Rotation sequence: yaw, pitch, roll [WRONG, DO NOT USE]
% phi_relative = atan(A(2,1)/A(1,1));
% theta_relative = atan(-A(3,1)/sqrt(1-(A(3,1))^2));
% psi_relative = atan(A(3,2)/A(3,3));

% Rotation sequence: roll, pitch, yaw [CORRECT, SEE 'Rotation_sequence_check.m']
% phi_relative = atan(-A(2,3)/A(3,3));
% theta_relative = atan(A(1,3)/sqrt(1-(A(1,3))^2));
% psi_relative = atan(-A(1,2)/A(1,1));

% phi_acm = atan(-Aa(2,3)/Aa(3,3));
% theta_acm = atan(Aa(1,3)/sqrt(1-(Aa(1,3))^2));
% psi_acm = atan(-Aa(1,2)/Aa(1,1));
% 
% phi_arm = atan(-Ar(2,3)/Ar(3,3));
% theta_arm = atan(Ar(1,3)/sqrt(1-(Ar(1,3))^2));
% psi_arm = atan(-Ar(1,2)/Ar(1,1));

% The rotation sequence of the model-arm gimbal is actually: yaw, pitch, roll
% psi_relative = atan(A(2,1)/A(1,1));
% theta_relative = atan(-A(3,1)/sqrt(1-(A(3,1))^2));
% phi_relative = atan(A(3,2)/A(3,3));
% 
% psi_acm = atan(Aa(2,1)/Aa(1,1));
% theta_acm = atan(-Aa(3,1)/sqrt(1-(Aa(3,1))^2));
% phi_acm = atan(Aa(3,2)/A(3,3));
% 
% psi_arm = atan(Ar(2,1)/Ar(1,1));
% theta_arm = atan(-Ar(3,1)/sqrt(1-(Ar(3,1))^2));
% phi_arm = atan(Ar(3,2)/Ar(3,3));
psi_relative = atan2(A(2,1),A(1,1));
theta_relative = atan2(-A(3,1),sqrt(1-(A(3,1))^2));
phi_relative = atan2(A(3,2),A(3,3));

psi_acm = atan2(Aa(2,1),Aa(1,1));
theta_acm = atan2(-Aa(3,1),sqrt(1-(Aa(3,1))^2));
phi_acm = atan2(Aa(3,2),A(3,3));

psi_arm = atan2(Ar(2,1),Ar(1,1));
theta_arm = atan2(-Ar(3,1),sqrt(1-(Ar(3,1))^2));
phi_arm = atan2(Ar(3,2),Ar(3,3));

== matlab function constraints_comparison_Corsair/Subsystem14/Physical deflections to virtual compensator deflections ==
  data: da_cmp output; servo1 input; de_cmp output; dr_cmp output; servo2 input; servo3 input; servo4 input
function [da_cmp, de_cmp, dr_cmp] = fcn(servo1,servo2,servo3,servo4)

s = [   servo1
        servo2
        servo3
        servo4  ];
    
A = [   1    1  -1   1
        1   -1  -1  -1
        1   -1   1  +1
        1    1   1  -1  ];
    
% NOTE: last column on matrix A is redundant to make a square matrix for
% inversion
    
d = A\s;

da_cmp = d(1);
de_cmp = d(2);
dr_cmp = d(3);

== matlab function constraints_comparison_Corsair/Integrator for velocity/MATLAB Function ==
  data: p_rig input; u_ini output; v_ini output; w_ini output; q_rig input; r_rig input; q1 input; qr input; p_acm input; q_dot output; q_acm input; r_acm input
function [u_ini,v_ini,w_ini,q_dot]= fcn(p_rig,q_rig,r_rig,q1,qr,p_acm,q_acm,r_acm)

% Initial position

% r = 0.8;
% 
% x_ini = r*cos(theta_rig);
% y_ini = 0;
% z_ini = -r*sin(theta_rig);
% 
% u_ini = q_rig*z_ini; 
% v_ini = 0;
% w_ini = -q_rig*x_ini;

% Initial position
x_ini = 0.95*0;
y_ini = 0;
z_ini = 0;

% Local velocities in body axes (Cook, pg.74)
u_ini_body = q_rig*z_ini - r_rig*y_ini;
v_ini_body = r_rig*x_ini - p_rig*z_ini;
w_ini_body = p_rig*y_ini - q_rig*x_ini;

q00 = qr(4);
q11 = qr(5);
q22 = qr(6);
q33 = qr(7);

E = [  -q11     q00      -q33     q22
        -q22     q33      q00      -q11
        -q33     -q22     q11      q00  ];
    
E_dash = [     -q11     q00      q33      -q22
                -q22     -q33     q00      q11
                -q33     q22      -q11     q00  ];

% Body to inertial axes
A = E*transpose(E_dash);

% Inertial axes velocity
V_inertial = A*[    u_ini_body  
                    v_ini_body  
                    w_ini_body      ];
                
u_ini = V_inertial(1);
v_ini = V_inertial(2);
w_ini = V_inertial(3);

q = [   q1(4)
        q1(5)
        q1(6)
        q1(7)    ];

Q = [   -q(2)   -q(3)   -q(4)
        q(1)    -q(4)   q(3)
        q(4)    q(1)    -q(2)
        -q(3)   q(2)    q(1)    ];

omega = [   p_acm
            q_acm
            r_acm       ];

q_dot = 0.5*Q*omega;

== matlab function constraints_comparison_Corsair/Integrator for position/MATLAB Function ==
  data: q input; x_ini output; y_ini output; z_ini output
function [x_ini,y_ini,z_ini]= fcn(q)

% Initial position

r = 0.8*0;

p = [   r
        0
        0   ];

q0 = q(1);
q1 = q(2);
q2 = q(3);
q3 = q(4);

E = [  -q1     q0      -q3     q2
       -q2     q3      q0      -q1
       -q3     -q2     q1      q0  ];
    
E_dash = [     -q1     q0      q3      -q2
               -q2     -q3     q0      q1
               -q3     q2      -q1     q0  ];
           
A = E*transpose(E_dash);

p_in = A*p;

x_ini = p_in(1);
y_ini = p_in(2);
z_ini = p_in(3);

== matlab function constraints_comparison_Corsair/Subsystem/HHIRM ==
  data: Aa input size=[1]; E_dasha input size=[1]; dail input; dele input; drud input; Fa output; M_dash_a output; CX output; CY output; CZ output
function [Fa,M_dash_a,CX,CY,CZ] = fcn(Aa,E_dasha,dail,dele,drud)

rho = 1.225;%1.218; % Density (kg/m^3)
% rho = 1.218; % Density (kg/m^3) Bristol

V_t = 30; % Tunnel windspeed (m/s)

%% Calculating angle of attack (alpha), sideslip (sideslip) and local angular velocities (p, q, r)

% Velocity of aircraft in inertial axes
V_a_dot_inertial = [    qa_dot(1)+V_t
                        qa_dot(2)
                        qa_dot(3)      ];

% Velocity of aircraft in body axes (vector_inertial = A * vector_body, where A is the transformation matrix)
V_a_dot_body = transpose(Aa)*V_a_dot_inertial;

% Magnitude of total local velocity vector
V = sqrt((V_a_dot_inertial(1))^2+(V_a_dot_inertial(2))^2+(V_a_dot_inertial(3))^2);

% Angle of attack (alpha)
alpha = atan2(V_a_dot_body(3),V_a_dot_body(1));

% Sideslip angle (beta)
beta = asin(V_a_dot_body(2)/V);

% Local angular velocities (p, q, r in body axes)
omega_dasha = 2*E_dasha*[	qa0_dot
                            qa1_dot
                            qa2_dot
                            qa3_dot     ];

p = omega_dasha(1);
q = omega_dasha(2);
r = omega_dasha(3);

%% Reference dimensions (Hawk)
c = 0.143;       % m
S = 0.084942;    % m^2
b = 0.594;       % m

% Reference dimensions (T-tail)
% c = 0.1417;       % m
% S = 0.1077;       % m^2
% b = 0.8967;       % m

%% Defining variables for HHIRM

ALPHA = alpha;
BETA = beta;
PW_UND=p*b/(2*V);
RW_UND=r*b/(2*V);
QW_UND=q*c/(2*V);

DELTA_e=dele;
DELTA_r=drud;
DELTA_a=dail;
DELTA_dh=0;

DELTA_pp=0;
DELTA_py=0;
DELTA_sp=0;
DELTA_sy=0;
tcs=1.;
tcp=1.;

KCX_tol=0;
KCY_tol=0;
KCZ_tol=0;
KCL_tol=0;
KCM_tol=0;
KCN_tol=0;

%% HHIRM

[CX]=acx(ALPHA,BETA,PW_UND,RW_UND,QW_UND,DELTA_e,...
		DELTA_dh,DELTA_a,DELTA_r,DELTA_pp,DELTA_py,...
		DELTA_sp,DELTA_sy,tcs,tcp,KCX_tol,KCY_tol,...
		KCZ_tol,KCL_tol,KCM_tol,KCN_tol);
    
[CY]=acy(ALPHA,BETA,PW_UND,RW_UND,QW_UND,DELTA_e,...
		DELTA_dh,DELTA_a,DELTA_r,DELTA_pp,DELTA_py,...
		DELTA_sp,DELTA_sy,tcs,tcp,KCX_tol,KCY_tol,...
		KCZ_tol,KCL_tol,KCM_tol,KCN_tol);

[CZ]=acz(ALPHA,BETA,PW_UND,RW_UND,QW_UND,DELTA_e,...
		DELTA_dh,DELTA_a,DELTA_r,DELTA_pp,DELTA_py,...
		DELTA_sp,DELTA_sy,tcs,tcp,KCX_tol,KCY_tol,...
		KCZ_tol,KCL_tol,KCM_tol,KCN_tol);
    
[CL]=acl(ALPHA,BETA,PW_UND,RW_UND,QW_UND,DELTA_e,...
		DELTA_dh,DELTA_a,DELTA_r,DELTA_pp,DELTA_py,...
		DELTA_sp,DELTA_sy,tcs,tcp,KCX_tol,KCY_tol,...
		KCZ_tol,KCL_tol,KCM_tol,KCN_tol);
    
[CM]=acm(ALPHA,BETA,PW_UND,RW_UND,QW_UND,DELTA_e,...
		DELTA_dh,DELTA_a,DELTA_r,DELTA_pp,DELTA_py,...
		DELTA_sp,DELTA_sy,tcs,tcp,KCX_tol,KCY_tol,...
		KCZ_tol,KCL_tol,KCM_tol,KCN_tol);
    
[CN]=acn(ALPHA,BETA,PW_UND,RW_UND,QW_UND,DELTA_e,...
		DELTA_dh,DELTA_a,DELTA_r,DELTA_pp,DELTA_py,...
		DELTA_sp,DELTA_sy,tcs,tcp,KCX_tol,KCY_tol,...
		KCZ_tol,KCL_tol,KCM_tol,KCN_tol);
    
%% Wind axes forces and moments
X=0.5*rho*V^2*S*CX;
Y=0.5*rho*V^2*S*CY;
Z=0.5*rho*V^2*S*CZ;

L=0.5*rho*V^2*S*b*CL;
M=0.5*rho*V^2*S*c*CM;
N=0.5*rho*V^2*S*b*CN;

F_wind = [  X
            Y
            Z   ];
        
M_wind = [  L
            M
            N   ];
        
%% Body to wind axes transformation
% According to Cook (page 21): (phi,theta,psi) = (0,alpha,-beta)
phi_w = 0;
theta_w = alpha;
psi_w = -beta;

% From NASA transformation equations:
theta1 = psi_w;
theta2 = theta_w;
theta3 = phi_w;

q0 = +sin(theta1/2)*sin(theta2/2)*sin(theta3/2)+cos(theta1/2)*cos(theta2/2)*cos(theta3/2);
q1 = -sin(theta1/2)*sin(theta2/2)*cos(theta3/2)+sin(theta3/2)*cos(theta1/2)*cos(theta2/2);
q2 = +sin(theta1/2)*sin(theta3/2)*cos(theta2/2)+sin(theta2/2)*cos(theta1/2)*cos(theta3/2);
q3 = +sin(theta1/2)*cos(theta2/2)*cos(theta3/2)-sin(theta2/2)*sin(theta3/2)*cos(theta1/2);

E = [  -q1     q0      -q3     q2
        -q2     q3      q0      -q1
        -q3     -q2     q1      q0  ];
    
E_dash = [     -q1     q0      q3      -q2
                -q2     -q3     q0      q1
                -q3     q2      -q1     q0  ];
            
A_b2w = E*transpose(E_dash); % Note: this matrx transforms from body to wind axes!

%% Body axes forces and moments
F_dash_a = transpose(A_b2w)*F_wind;
M_dash_a = transpose(A_b2w)*M_wind;

%% Inertial axes moments
Fa = Aa*F_dash_a;

== matlab function constraints_comparison_Corsair/Subsystem/MATLAB Function3 ==
  data: V0 output size=[1]; qa input size=[7,1]; alpha output size=[1]; beta output; qa_dot input size=[7,1]; w_dot output size=[1]; q output size=[1]; qa_dot_dot input; Vt input; Va output; qa_wind output
function [V0,alpha,beta,w_dot,q,Va,qa_wind] = fcn(qa,qa_dot,qa_dot_dot,Vt)
  
Ra1 = qa(1);
Ra2 = qa(2);
Ra3 = qa(3);
qa0 = qa(4);
qa1 = qa(5);
qa2 = qa(6);
qa3 = qa(7);

Ra1_dot = qa_dot(1);
Ra2_dot = qa_dot(2);
Ra3_dot = qa_dot(3);
qa0_dot = qa_dot(4);
qa1_dot = qa_dot(5);
qa2_dot = qa_dot(6);
qa3_dot = qa_dot(7);

Ra1_dot_dot = qa_dot_dot(1);
Ra2_dot_dot = qa_dot_dot(2);
Ra3_dot_dot = qa_dot_dot(3);
qa0_dot_dot = qa_dot_dot(4);
qa1_dot_dot = qa_dot_dot(5);
qa2_dot_dot = qa_dot_dot(6);
qa3_dot_dot = qa_dot_dot(7);

% Transformation matrices
Ea = [  -qa1     qa0      -qa3     qa2
        -qa2     qa3      qa0      -qa1
        -qa3     -qa2     qa1      qa0  ];
    
E_dasha = [     -qa1     qa0      qa3      -qa2
                -qa2     -qa3     qa0      qa1
                -qa3     qa2      -qa1     qa0  ];

Aa = Ea*transpose(E_dasha);

% Wind tunnel velocity vector
Vtt = [  Vt
         0   
         0   ];

% Velocity vector of aircraft model in inertial frame of reference
Va = [  Ra1_dot
        Ra2_dot
        Ra3_dot	];

% Total velocity vector of aircraft model in body frame of reference
Va_dash = transpose(Aa)*(Va + Vtt);

% Magnitude of total local velocity vector
V0 = sqrt((Va_dash(1))^2+(Va_dash(2))^2+(Va_dash(3))^2);

% Angle of attack
alpha = atan2(Va_dash(3),Va_dash(1));

% Acceleration in body frame
a_dash = transpose(Aa)*[    Ra1_dot_dot
                            Ra2_dot_dot
                            Ra3_dot_dot     ];

% Acceleration in z-direction body frame
w_dot = a_dash(3);

% Sideslip angle [CHECK SIGN]
beta = asin(Va_dash(2)/V0);

% Local angular velocities (body axes)
omega_dasha = 2*E_dasha*[	qa0_dot
                            qa1_dot
                            qa2_dot
                            qa3_dot     ];
                        
% Pitch rate (body axes)
q = omega_dasha(2);

%% Calculating angular rates in wind axes

phi = 0;
theta = alpha;
psi = -beta;

theta1 = psi;
theta2 = theta;
theta3 = phi;

q0 = +sin(theta1/2)*sin(theta2/2)*sin(theta3/2)+cos(theta1/2)*cos(theta2/2)*cos(theta3/2);
q1 = -sin(theta1/2)*sin(theta2/2)*cos(theta3/2)+sin(theta3/2)*cos(theta1/2)*cos(theta2/2);
q2 = +sin(theta1/2)*sin(theta3/2)*cos(theta2/2)+sin(theta2/2)*cos(theta1/2)*cos(theta3/2);
q3 = +sin(theta1/2)*cos(theta2/2)*cos(theta3/2)-sin(theta2/2)*sin(theta3/2)*cos(theta1/2);

% E = [  -q1     q0      -q3     q2
%         -q2     q3      q0      -q1
%         -q3     -q2     q1      q0  ];
%     
% E_dash = [     -q1     q0      q3      -q2
%                 -q2     -q3     q0      q1
%                 -q3     q2      -q1     q0  ];
%             
%  A_b2w = E*transpose(E_dash); % body axes to inertial/wind axes transformation

qa_wind = [ q0
            q1
            q2
            q3	];

== matlab function constraints_comparison_Corsair/Subsystem/Wind axes angular rates calculation ==
  data: qa input size=[7,1]; p output size=[1]; q output size=[1]; qa_wind_dot input size=[4,1]; r output size=[1]; A_b2w output
function [p,q,r,A_b2w] = fcn(qa,qa_wind_dot)

qa0 = qa(4);
qa1 = qa(5);
qa2 = qa(6);
qa3 = qa(7);

qa0_dot = qa_wind_dot(1);
qa1_dot = qa_wind_dot(2);
qa2_dot = qa_wind_dot(3);
qa3_dot = qa_wind_dot(4);

% Transformation matrices
Ea = [  -qa1     qa0      -qa3     qa2
        -qa2     qa3      qa0      -qa1
        -qa3     -qa2     qa1      qa0  ];
    
E_dasha = [     -qa1     qa0      qa3      -qa2
                -qa2     -qa3     qa0      qa1
                -qa3     qa2      -qa1     qa0  ];

A_b2w = Ea*transpose(E_dasha); % body axes to inertial/wind axes transformation

new_E_dasha = Ea;

% Local angular velocities (wind axes)
omega_dasha = 2*E_dasha*[	qa0_dot
                           	qa1_dot
                           	qa2_dot
                           	qa3_dot     ];
                        
% Pitch rate (body axes)
p = omega_dasha(1); % rad/s
q = omega_dasha(2); % rad/s
r = omega_dasha(3); % rad/s

== matlab function constraints_comparison_Corsair/Subsystem14/Subsystem10/MATLAB Function ==
  data: p_rig input; u_ini output; v_ini output; w_ini output; q_rig input; r_rig input; q1 input; q_dot output
function [u_ini,v_ini,w_ini,q_dot]= fcn(p_rig,q_rig,r_rig, q1)

% Initial position

% x = 0.8;
% z = 0.3183;
% 
% theta_pos = atan(z/x) - theta_rig;
% r = sqrt(x^2+z^2);
% 
% u_ini = q_rig*r*sin(theta_pos); 
% v_ini = 0;
% w_ini = -q_rig*r*cos(theta_pos);
% 
% q = [   q1(4)
%         q1(5)
%         q1(6)
%         q1(7)    ];
% 
% Q = [   -q(2)   -q(3)   -q(4)
%         q(1)    -q(4)   q(3)
%         q(4)    q(1)    -q(2)
%         -q(3)   q(2)    q(1)    ];
% 
% omega = [   0
%             q_rig
%             0       ];
% 
% q_dot = 0.5*Q*omega;

% Initial position
x_ini = 0.95;
y_ini = 0;
z_ini = 0.3183;

% Local velocities in body axes (Cook, pg.74)
u_ini_body = q_rig*z_ini - r_rig*y_ini;
v_ini_body = r_rig*x_ini - p_rig*z_ini;
w_ini_body = p_rig*y_ini - q_rig*x_ini;

q00 = q1(4);
q11 = q1(5);
q22 = q1(6);
q33 = q1(7);

E = [  -q11     q00      -q33     q22
        -q22     q33      q00      -q11
        -q33     -q22     q11      q00  ];
    
E_dash = [     -q11     q00      q33      -q22
                -q22     -q33     q00      q11
                -q33     q22      -q11     q00  ];

% Body to inertial axes
A = E*transpose(E_dash);

% Inertial axes velocity
V_inertial = A*[    u_ini_body  
                    v_ini_body  
                    w_ini_body      ];
                
u_ini = V_inertial(1);
v_ini = V_inertial(2);
w_ini = V_inertial(3);

q = [   q1(4)
        q1(5)
        q1(6)
        q1(7)    ];

Q = [   -q(2)   -q(3)   -q(4)
        q(1)    -q(4)   q(3)
        q(4)    q(1)    -q(2)
        -q(3)   q(2)    q(1)    ];

omega = [   p_rig
            q_rig
            r_rig       ];

q_dot = 0.5*Q*omega;
